simulink model "FPFFT_001"  (R2021a)
settings: Solver=VariableStepAuto  StartTime=0.0  StopTime=10.0  RelTol=1e-3
InitFcn:
  | SSR=2;
undefined symbols (not defined in the file): xc7vx485tffg1157
libraries: hdlSSR x13, hdlBasic x4, vmcUtilities x1
settings Model: Creator=catalinb  LastModifiedBy=catalinb

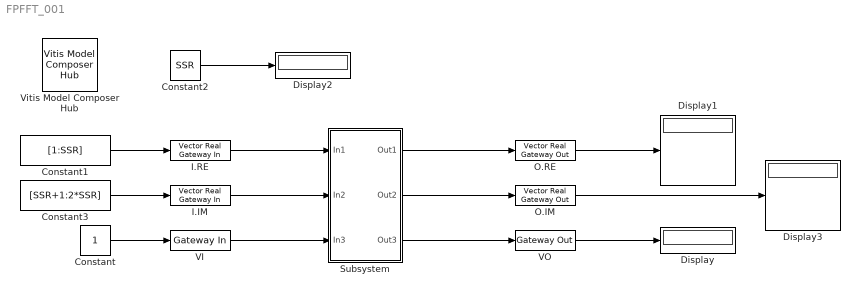
== system FPFFT_001 ==
  Constant : Constant  SampleTime=-1
  Constant1 : Constant  Value=[1:SSR]  SampleTime=-1
  Constant2 : Constant  Value=SSR  SampleTime=-1
  Constant3 : Constant  Value=[SSR+1:2*SSR]  SampleTime=-1
  Display{,1..3} (4 alike) : Display
  I.IM : hdlSSR/Vector Real Gateway In  gui_display_data_type=Floating-point  arith_type=Floating-point  n_bits=16  bin_pt=14  preci_type=Single  exp_width=8  frac_width=24  quantization="Round  (unbiased: +/- Inf)"  overflow=Saturate  period=1  sg_ssr=SSR  UseAsADC=off  ADCChannel='1'  interface=None  automatic_assignment=on  address_offset=hex2dec('00')  intf_name=''  intf_description=''  default_value=0  timing_constraint=None  locs_specified=off  LOCs={}  io_standard={}  inherit_from_input=off  hdl_port=on  interface_prev=1  block_type=realgatewayin_ssr  XmcBlockStatus=1  sg_ssr_prev=2  maskContainerNames=group4  block_width_w=590  block_height_w=670  block_width=640  block_height=850
  I.RE : hdlSSR/Vector Real Gateway In  gui_display_data_type=Floating-point  arith_type=Floating-point  n_bits=16  bin_pt=14  preci_type=Single  exp_width=8  frac_width=24  quantization="Round  (unbiased: +/- Inf)"  overflow=Saturate  period=1  sg_ssr=SSR  UseAsADC=off  ADCChannel='1'  interface=None  automatic_assignment=on  address_offset=hex2dec('00')  intf_name=''  intf_description=''  default_value=0  timing_constraint=None  locs_specified=off  LOCs={}  io_standard={}  inherit_from_input=off  hdl_port=on  interface_prev=1  block_type=realgatewayin_ssr  XmcBlockStatus=1  sg_ssr_prev=2  maskContainerNames=group4  block_width_w=590  block_height_w=670  block_width=640  block_height=850
  O.IM : hdlSSR/Vector Real Gateway Out  inherit_from_input=off  hdl_port=on  sg_ssr=SSR  rows=1  columns=1  UseAsDAC=off  DACChannel='1'  interface=None  automatic_assignment=on  address_offset=hex2dec('00')  intf_name=''  intf_description=''  timing_constraint=None  locs_specified=off  LOCs={}  io_standard={}  block_type=realgatewayout_ssr  XmcBlockStatus=1  sg_ssr_prev=2  maskContainerNames=group4  block_width_w=590  block_height_w=620  block_width=620  block_height=750
  O.RE : hdlSSR/Vector Real Gateway Out  inherit_from_input=off  hdl_port=on  sg_ssr=SSR  rows=1  columns=1  UseAsDAC=off  DACChannel='1'  interface=None  automatic_assignment=on  address_offset=hex2dec('00')  intf_name=''  intf_description=''  timing_constraint=None  locs_specified=off  LOCs={}  io_standard={}  block_type=realgatewayout_ssr  XmcBlockStatus=1  sg_ssr_prev=2  maskContainerNames=group4  block_width_w=590  block_height_w=620  block_width=620  block_height=750
  Subsystem : Subsystem  mask{SSR=SSR}
  VI : hdlBasic/Gateway In  gui_display_data_type=Boolean  arith_type=Boolean  n_bits=16  bin_pt=14  preci_type=Single  exp_width=8  frac_width=24  rows=1  columns=1  quantization="Round  (unbiased: +/- Inf)"  overflow=Saturate  period=1  UseAsADC=off  ADCChannel='1'  interface=None  automatic_assignment=on  address_offset=hex2dec('00')  intf_name=''  intf_description=''  default_value=0  timing_constraint=None  locs_specified=off  LOCs={}  io_standard={}  inherit_from_input=off  hdl_port=on  XmcBlockStatus=1  maskContainerNames=group4  block_type=gatewayin  block_config=sysgen:gateway_in_config  block_width_w=590  block_height_w=620  block_width=640  block_height=850
  VO : hdlBasic/Gateway Out  inherit_from_input=off  hdl_port=on  rows=1  columns=1  UseAsDAC=off  DACChannel='1'  interface=None  automatic_assignment=on  address_offset=hex2dec('00')  intf_name=''  intf_description=''  timing_constraint=None  locs_specified=off  LOCs={}  io_standard={}  XmcBlockStatus=1  maskContainerNames=group4  block_type=gatewayout  block_config=sysgen:gateway_out_config  block_width_w=590  block_height_w=620  block_width=620  block_height=750
  Vitis Model Composer Hub : vmcUtilities/Vitis Model Composer Hub  Tag=genX  CodeGeneration=off  SubsystemName=<enter or select subsystem name>  TargetDirectory=./code  ExportType=HLS C++ code  IpVendor=xilinx.com  IpLibrary=hls  IpVersion=1.0  IpHWLanguage=Verilog  AieCompilerOptions={}  CreateTestbench=off  TestbenchStackSize=10  RunAieSim=off  AieSimTimeout=50000  RunAieSimProfiling=off  LaunchVitisAnalyzer=off  PlotOutput=off  RunX86Sim=off  X86SimTimeout=10  GenHwImage=off  PlatformType=Not Specified  HwSystemType=Baremetal  HwValidationTarget=hw  ProjDevice=xc7vx485tffg1157-3  ProjDevicePart=xc7vx485tffg1157-3  SamplePeriod=-1  ClockFrequency=200  DataPathParallelism=1  xilinxfamily=virtex7  part=xc7vx485t  speed=-3  package=ffg1157  directory=./netlist  testbench=off  incr_netlist=off  synthesis_tool=Vivado  clock_wrapper=Clock Enables  dbl_ovrd=According to Block Masks  dcm_input_clock_period=10  sysclk_period=1  simulink_period=1  eval_field=0
  wires:
  Constant/1 -> VI/1
  VO/1 -> Display/1
  O.RE/1 -> Display1/1
  Constant1/1 -> I.RE/1
  Constant2/1 -> Display2/1
  Constant3/1 -> I.IM/1
  O.IM/1 -> Display3/1
  I.RE/1 -> Subsystem/1(In1)
  I.IM/1 -> Subsystem/2(In2)
  VI/1 -> Subsystem/3(In3)
  Subsystem/1(Out1) -> O.RE/1
  Subsystem/2(Out2) -> O.IM/1
  Subsystem/3(Out3) -> VO/1

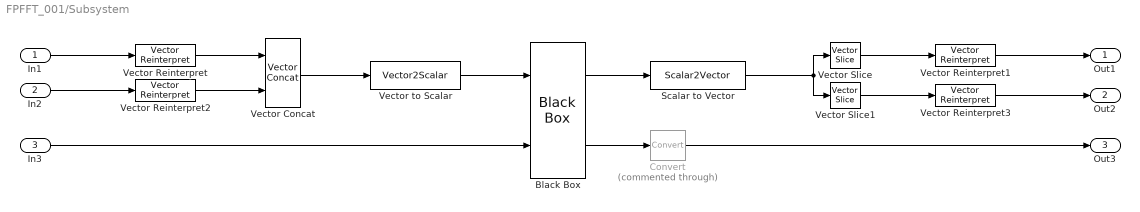
== system FPFFT_001/Subsystem ==
  In1 : Inport
  In2 : Inport  Port=2
  In3 : Inport  Port=3
  Black Box : hdlBasic/Black Box  init_code=WRAPPER_PARFFT2_config  sim_method=Vivado Simulator  verbose=off  XmcBlockStatus=1  maskContainerNames=group1  block_type=blackbox2  block_config=sysgen:black_box_config
  Convert : hdlBasic/Convert  Commented=through  gui_display_data_type=Boolean  arith_type=Boolean  n_bits=16  bin_pt=14  float_type=Single  exp_bits=8  fraction_bits=24  quantization=Truncate  overflow=Wrap  en=off  latency=0  pipeline=off  XmcBlockStatus=1  maskContainerNames=group2  block_type=convert  block_config=sysgen:Convert_config
  Scalar to Vector : hdlSSR/Scalar2Vector  Width=2*32  sg_ssr=SSR  block_type=scalar2vector_ssr  XmcBlockStatus=1  sg_ssr_prev=2  maskContainerNames=group1
      settings: SourceProductName=Xilinx SSR Blockset
  Vector Concat : hdlSSR/Vector Concat  num_inputs=2  sg_ssr=SSR  num_inputs_prev=2  block_type=concat_ssr  XmcBlockStatus=1  sg_ssr_prev=2  maskContainerNames=group1
  Vector Reinterpret : hdlSSR/Vector Reinterpret  force_arith_type=on  arith_type=Unsigned  force_bin_pt=on  bin_pt=0  sg_ssr=SSR  block_type=reinterpret_ssr  XmcBlockStatus=1  sg_ssr_prev=2  maskContainerNames=group1
  Vector Reinterpret1 : hdlSSR/Vector Reinterpret  force_arith_type=on  arith_type=Floating-point  force_bin_pt=on  bin_pt=24  sg_ssr=SSR  block_type=reinterpret_ssr  XmcBlockStatus=1  sg_ssr_prev=2  maskContainerNames=group1
  Vector Reinterpret2 : hdlSSR/Vector Reinterpret  force_arith_type=on  arith_type=Unsigned  force_bin_pt=on  bin_pt=0  sg_ssr=SSR  block_type=reinterpret_ssr  XmcBlockStatus=1  sg_ssr_prev=2  maskContainerNames=group1
  Vector Reinterpret3 : hdlSSR/Vector Reinterpret  force_arith_type=on  arith_type=Floating-point  force_bin_pt=on  bin_pt=24  sg_ssr=SSR  block_type=reinterpret_ssr  XmcBlockStatus=1  sg_ssr_prev=2  maskContainerNames=group1
  Vector Slice : hdlSSR/Vector Slice  nbits=32  boolean_output=off  mode=Lower Bit Location + Width  bit1=0  base1=MSB of Input  bit0=32  base0=LSB of Input  sg_ssr=SSR  block_type=slice_ssr  XmcBlockStatus=1  sg_ssr_prev=2  maskContainerNames=group1
  Vector Slice1 : hdlSSR/Vector Slice  nbits=32  boolean_output=off  mode=Lower Bit Location + Width  bit1=0  base1=MSB of Input  bit0=0  base0=LSB of Input  sg_ssr=SSR  block_type=slice_ssr  XmcBlockStatus=1  sg_ssr_prev=2  maskContainerNames=group1
  Vector to Scalar : hdlSSR/Vector2Scalar  sg_ssr=SSR  block_type=vector2scalar_ssr  XmcBlockStatus=1  sg_ssr_prev=2  maskContainerNames=group1
      settings: SourceProductName=Xilinx SSR Blockset
  Out1 : Outport
  Out2 : Outport  Port=2
  Out3 : Outport  Port=3
  wires:
  Vector Slice/1 -> Vector Reinterpret1/1
  In1/1 -> Vector Reinterpret/1
  Vector Slice1/1 -> Vector Reinterpret3/1
  Vector Reinterpret/1 -> Vector Concat/1
  Scalar to Vector/1 -> Vector Slice1/1, Vector Slice/1
  Vector Reinterpret2/1 -> Vector Concat/2
  Vector Concat/1 -> Vector to Scalar/1
  Vector to Scalar/1 -> Black Box/1
  In2/1 -> Vector Reinterpret2/1
  Black Box/1 -> Scalar to Vector/1
  Vector Reinterpret1/1 -> Out1/1
  Vector Reinterpret3/1 -> Out2/1
  In3/1 -> Black Box/2
  Black Box/2 -> Convert/1
  Convert/1 -> Out3/1
